simulink model "Motor_model"  (R2025b)
settings: Solver=ode45  StartTime=0.0  StopTime=3  MaxStep=1e-5  RelTol=1e-5
libraries: simulink x2
settings Model: Creator=Matlab  LastModifiedBy=noeliarosales
settings ModelReferenceCC: EnableRefExpFcnMdlSchedulingChecks=on
settings RTWCC: GPUComputeCapability=3.5

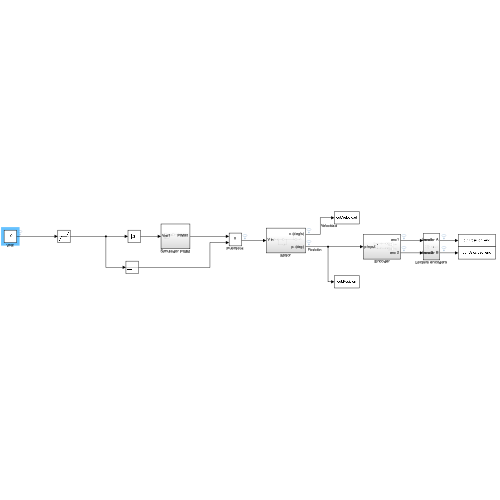
[thumbnail: Simulink's stored preview of the top-level diagram]
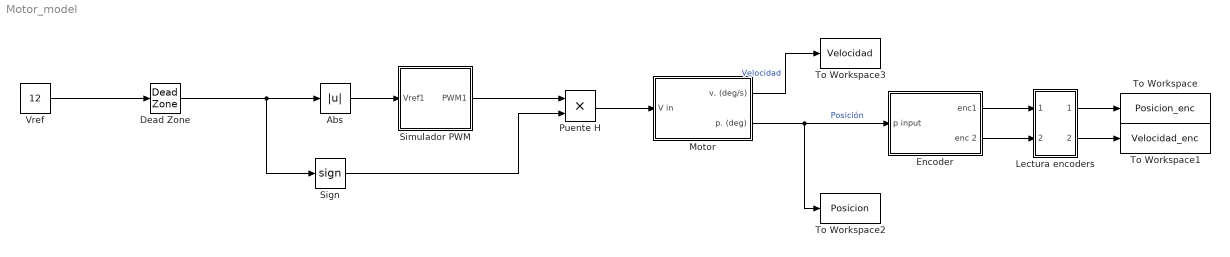
== system Motor_model ==
  " Encoder" : Subsystem
  Abs : Abs  SaturateOnIntegerOverflow=off
  Dead Zone : DeadZone
  Lectura encoders : Subsystem
  Motor : Subsystem
  Puente H : Product
  Sign : Signum
  Simulador PWM : Subsystem
  To Workspace : ToWorkspace  VariableName=Posicion_enc  SaveFormat=Timeseries  SampleTime=-1
  To Workspace1 : ToWorkspace  VariableName=Velocidad_enc  SaveFormat=Timeseries  SampleTime=-1
  To Workspace2 : ToWorkspace  VariableName=Posicion  SaveFormat=Timeseries  SampleTime=-1
  To Workspace3 : ToWorkspace  VariableName=Velocidad  SaveFormat=Timeseries  SampleTime=-1
  Vref : Constant  Value=12
  wires:
  Vref/1 -> Dead Zone/1
  Sign/1 -> Puente H/2
  Puente H/1 -> Motor/1(V in)
  Motor/1(v. (deg/s)) -> To Workspace3/1  "Velocidad"
  Dead Zone/1 -> Sign/1, Abs/1
  Abs/1 -> Simulador PWM/1(Vref1)
  Simulador PWM/1(PWM1) -> Puente H/1
  Motor/2(p. (deg)) -> To Workspace2/1, " Encoder"/1(p input)  "Posición"
  " Encoder"/1(enc1) -> Lectura encoders/1(enc1)
  " Encoder"/2(enc 2) -> Lectura encoders/2(enc 2)
  Lectura encoders/1(Encoder A) -> To Workspace/1
  Lectura encoders/2(Encoder B) -> To Workspace1/1

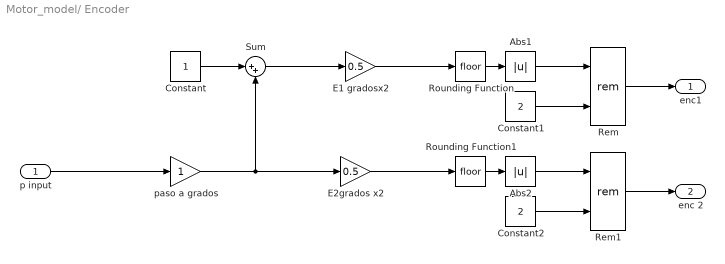
== system Motor_model/ Encoder ==
  p input : Inport
  Abs1 : Abs  SaturateOnIntegerOverflow=off
  Abs2 : Abs  SaturateOnIntegerOverflow=off
  Constant : Constant
  Constant1 : Constant  Value=2
  Constant2 : Constant  Value=2
  E1 gradosx2 : Gain  Gain=0.5
  E2grados x2 : Gain  Gain=0.5
  Rem : Math  Operator=rem
  Rem1 : Math  Operator=rem
  Rounding Function : Rounding
  Rounding Function1 : Rounding
  Sum : Sum  Inputs=|++
  paso a grados : Gain
  enc1 : Outport
  enc 2 : Outport  Port=2
  wires:
  paso a grados/1 -> E2grados x2/1, Sum/2
  p input/1 -> paso a grados/1
  Sum/1 -> E1 gradosx2/1
  Constant/1 -> Sum/1
  E1 gradosx2/1 -> Rounding Function/1
  E2grados x2/1 -> Rounding Function1/1
  Rounding Function/1 -> Abs1/1
  Abs1/1 -> Rem/1
  Constant1/1 -> Rem/2
  Rounding Function1/1 -> Abs2/1
  Abs2/1 -> Rem1/1
  Constant2/1 -> Rem1/2
  Rem1/1 -> enc 2/1
  Rem/1 -> enc1/1

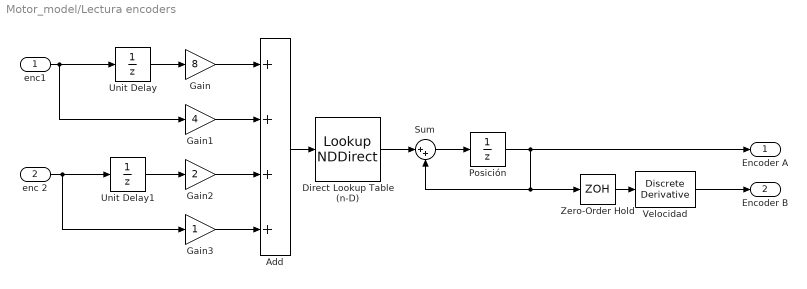
== system Motor_model/Lectura encoders ==
  enc1 : Inport
  enc 2 : Inport  Port=2
  Add : Sum  Inputs=++++  OutDataTypeStr=double
  Direct Lookup Table (n-D) : LookupNDDirect  NumberOfTableDimensions=1  Table=[0,-1,1,0,1,0,0,-1,-1,0,0,1,0,1,-1,0]
  Gain : Gain  Gain=8
  Gain1 : Gain  Gain=4
  Gain2 : Gain  Gain=2
  Gain3 : Gain
  Posición : UnitDelay  SampleTime=-1  HasFrameUpgradeWarning=on
  Sum : Sum  Inputs=|++
  Unit Delay : UnitDelay  SampleTime=-1  HasFrameUpgradeWarning=on
  Unit Delay1 : UnitDelay  SampleTime=-1  HasFrameUpgradeWarning=on
  Velocidad : simulink/Discrete/Discrete Derivative  gainval=1.0  ICPrevScaledInput=0.0  OutMin=[]  OutMax=[]  OutDataType=fixdt(1, 16)  OutScaling=2^-10  DoSatur=off
  Zero-Order Hold : ZeroOrderHold  SampleTime=0.0001
  Encoder A : Outport
  Encoder B : Outport  Port=2
  wires:
  Add/1 -> Direct Lookup Table (n-D)/1
  Unit Delay/1 -> Gain/1
  enc 2/1 -> Gain3/1, Unit Delay1/1
  Sum/1 -> Posición/1
  Direct Lookup Table (n-D)/1 -> Sum/1
  Posición/1 -> Encoder A/1, Sum/2, Zero-Order Hold/1
  Zero-Order Hold/1 -> Velocidad/1
  Gain1/1 -> Add/2
  Gain3/1 -> Add/4
  Gain2/1 -> Add/3
  Unit Delay1/1 -> Gain2/1
  enc1/1 -> Unit Delay/1, Gain1/1
  Gain/1 -> Add/1
  Velocidad/1 -> Encoder B/1

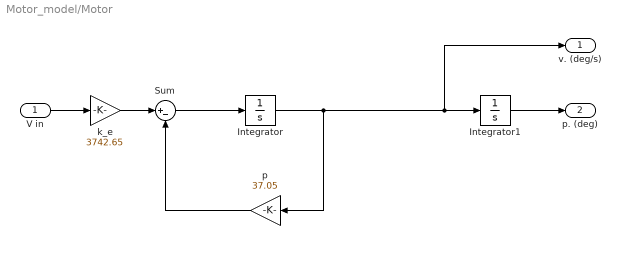
== system Motor_model/Motor ==
  V in : Inport
  Integrator : Integrator
  Integrator1 : Integrator
  Sum : Sum  Inputs=|+-
  k_e : Gain  Gain=3742.65
  p : Gain  Gain=37.05
  v. (deg/s) : Outport
  p. (deg) : Outport  Port=2
  wires:
  p/1 -> Sum/2
  k_e/1 -> Sum/1
  Integrator/1 -> v. (deg/s)/1, Integrator1/1, p/1
  Integrator1/1 -> p. (deg)/1
  V in/1 -> k_e/1
  Sum/1 -> Integrator/1

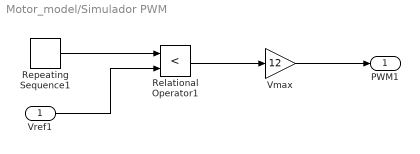
== system Motor_model/Simulador PWM ==
  Vref1 : Inport
  Relational Operator1 : RelationalOperator  Operator=<  OutDataTypeStr=boolean  RndMeth=Simplest  InputSameDT=off
  Repeating Sequence1 : simulink/Sources/Repeating Sequence  rep_seq_t=linspace(0,0.001,100)  rep_seq_y=linspace(0,12,100)
  Vmax : Gain  Gain=12
  PWM1 : Outport
  wires:
  Relational Operator1/1 -> Vmax/1
  Vmax/1 -> PWM1/1
  Vref1/1 -> Relational Operator1/2
  Repeating Sequence1/1 -> Relational Operator1/1
